simulink subsystem "controlador_clase"  (R2023b)
settings: Solver=VariableStepAuto  StartTime=0.0  StopTime=10.0  RelTol=1e-3
settings Model: Creator=Usuario_UMA  LastModifiedBy=Usuario_UMA

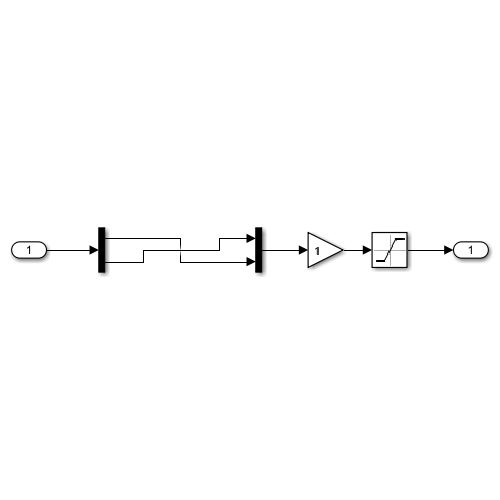
[thumbnail: Simulink's stored preview of the top-level diagram]
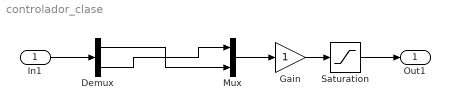
== system controlador_clase ==
  In1 : Inport
  Demux : Demux  Outputs=2
  Gain : Gain
  Mux : Mux  Inputs=2
  Saturation : Saturate  UpperLimit=100  LowerLimit=0
  Out1 : Outport
  wires:
  Saturation/1 -> Out1/1
  Demux/1 -> Mux/2
  Mux/1 -> Gain/1
  Demux/2 -> Mux/1
  Gain/1 -> Saturation/1
  In1/1 -> Demux/1
